simulink model "bille_synthese_RST"  (R2019a)
settings: Solver=VariableStepAuto  StartTime=0.0  StopTime=20  RelTol=1e-3
values from neighbouring files (symbols this model uses):
  f = 7E-5    (= 7e-05)    [BallOnBeam.m]
  J = 4.6E-5    (= 4.6e-05)    [BallOnBeam.m]
  k = 0.026    [BallOnBeam.m]
  k1 = 7    [BallOnBeam.m]
  k2 = 28.65    [BallOnBeam.m]
  k3 = 0.0159    [BallOnBeam.m]
  kb = 6.1    [BallOnBeam.m]
  ki = 1.6    [BallOnBeam.m]
  kp = nm*J*wndes^2/(k2*k*ki)    (= 27.0462934428)    [BallOnBeam.m]
  kpi = rm*tii*ki/taudesi    (= 1.6)    [BallOnBeam.m]
  kv = (2*xides*J*wndes - f)/(kp*ki*k*k3)    (= 0.093347474441)    [BallOnBeam.m]
  lm = 0.001    [BallOnBeam.m]
  nm = 960    [BallOnBeam.m]
  r0 = x(3)    [BallOnBeam.m]
  r1 = x(4)    [BallOnBeam.m]
  r2 = x(5)    [BallOnBeam.m]
  rm = 0.33    [BallOnBeam.m]
  s1 = x(2)    [BallOnBeam.m]
  T = r0 + r1 + r2    [BallOnBeam.m]
  Te = 0.2    [BallOnBeam.m]
  tii = 0.5*lm/rm    (= 0.00151515151515)    [BallOnBeam.m]
settings Model: Creator=DELL  LastModifiedBy=DELL

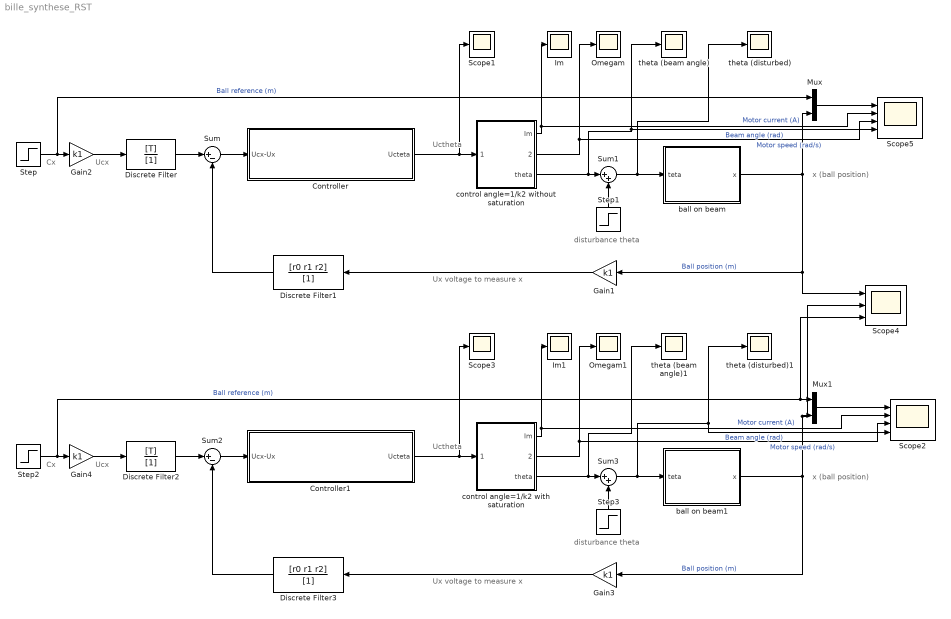
== system bille_synthese_RST ==
  note: disturbance theta
  note: Uctheta
  note: Ux voltage to measure x
  note: x (ball position)
  note: Cx
  note: Ucx
  note: Ux voltage to measure x
  note: Cx
  note: Uctheta
  note: Ucx
  note: disturbance theta
  note: x (ball position)
  Controller : Subsystem
  Controller1 : Subsystem
  Discrete Filter : DiscreteFilter  Numerator=[T]  Denominator=[1]
  Discrete Filter1 : DiscreteFilter  Numerator=[r0 r1 r2]  Denominator=[1]
  Discrete Filter2 : DiscreteFilter  Numerator=[T]  Denominator=[1]
  Discrete Filter3 : DiscreteFilter  Numerator=[r0 r1 r2]  Denominator=[1]
  Gain{1..4} (4 alike) : Gain  Gain=k1  SaturateOnIntegerOverflow=on  OutDataTypeStr=Inherit: Same as input  ParamDataTypeStr=Inherit: Same as input
  Im : Scope
  Im1 : Scope
  Mux : Mux  Inputs=2
  Mux1 : Mux  Inputs=2
  Omegam : Scope
  Omegam1 : Scope
  Scope1 : Scope
  Scope2 : Scope  NumInputPorts=4
  Scope3 : Scope
  Scope4 : Scope  NumInputPorts=3
  Scope5 : Scope  NumInputPorts=4
  Step : Step  After=0.1  SampleTime=0
  Step1 : Step  Time=10  After=1*pi/180  SampleTime=0
  Step2 : Step  After=0.1  SampleTime=0
  Step3 : Step  Time=10  After=1*pi/180  SampleTime=0
  Sum : Sum  Inputs=|+-  SaturateOnIntegerOverflow=on  InputSameDT=on  OutDataTypeStr=Inherit: Same as first input
  Sum1 : Sum  Inputs=|++  SaturateOnIntegerOverflow=on  InputSameDT=on  OutDataTypeStr=Inherit: Same as first input
  Sum2 : Sum  Inputs=|+-  SaturateOnIntegerOverflow=on  InputSameDT=on  OutDataTypeStr=Inherit: Same as first input
  Sum3 : Sum  Inputs=|++  SaturateOnIntegerOverflow=on  InputSameDT=on  OutDataTypeStr=Inherit: Same as first input
  ball on beam : Subsystem
  ball on beam1 : Subsystem
  control angle=1/k2 with saturation : Subsystem
  "control angle=1/k2 without saturation " : Subsystem
  theta (beam angle) : Scope
  theta (beam angle)1 : Scope
  theta (disturbed) : Scope
  theta (disturbed)1 : Scope
  wires:
  Sum1/1 -> theta (disturbed)/1, ball on beam/1(teta)
  "control angle=1/k2 without saturation "/2(omega) -> Omegam/1, Scope5/3  "Motor speed (rad/s)"
  Mux/1 -> Scope5/1
  "control angle=1/k2 without saturation "/3(theta) -> theta (beam angle)/1, Scope5/4, Sum1/1  "Beam angle (rad)"
  Step1/1 -> Sum1/2
  ball on beam/1(x) -> Scope4/1, Gain1/1, Mux/2  "Ball position (m)"
  Gain2/1 -> Discrete Filter/1
  Step/1 -> Mux/1, Gain2/1  "Ball reference (m)"
  Gain1/1 -> Discrete Filter1/1
  "control angle=1/k2 without saturation "/1(Im) -> Im/1, Scope5/2  "Motor current (A)"
  Discrete Filter/1 -> Sum/1
  Discrete Filter1/1 -> Sum/2
  Sum/1 -> Controller/1(Ucx-Ux)
  Controller/1(Ucteta) -> Scope1/1, "control angle=1/k2 without saturation "/1(Uctheta)
  control angle=1/k2 with saturation/3(theta) -> theta (beam angle)1/1, Sum3/1
  Sum2/1 -> Controller1/1(Ucx-Ux)
  Step3/1 -> Sum3/2
  Controller1/1(Ucteta) -> Scope3/1, control angle=1/k2 with saturation/1(Uctheta)
  Step2/1 -> Scope4/3, Mux1/1, Gain4/1  "Ball reference (m)"
  ball on beam1/1(x) -> Gain3/1, Scope4/2, Mux1/2  "Ball position (m)"
  Mux1/1 -> Scope2/1
  Sum3/1 -> theta (disturbed)1/1, Scope2/4, ball on beam1/1(teta)  "Beam angle (rad)"
  Discrete Filter3/1 -> Sum2/2
  Gain4/1 -> Discrete Filter2/1
  Gain3/1 -> Discrete Filter3/1
  control angle=1/k2 with saturation/2(omega) -> Omegam1/1, Scope2/3  "Motor speed (rad/s)"
  Discrete Filter2/1 -> Sum2/1
  control angle=1/k2 with saturation/1(Im) -> Im1/1, Scope2/2  "Motor current (A)"

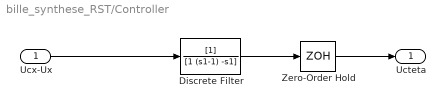
== system bille_synthese_RST/Controller ==
  Ucx-Ux : Inport
  Discrete Filter : DiscreteFilter  Denominator=[1 (s1-1) -s1]  SampleTime=Te
  Zero-Order Hold : ZeroOrderHold  SampleTime=-1
  Ucteta : Outport
  wires:
  Zero-Order Hold/1 -> Ucteta/1
  Discrete Filter/1 -> Zero-Order Hold/1
  Ucx-Ux/1 -> Discrete Filter/1

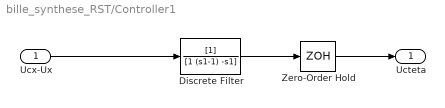
== system bille_synthese_RST/Controller1 ==
  Ucx-Ux : Inport
  Discrete Filter : DiscreteFilter  Denominator=[1 (s1-1) -s1]  SampleTime=Te
  Zero-Order Hold : ZeroOrderHold  SampleTime=-1
  Ucteta : Outport
  wires:
  Zero-Order Hold/1 -> Ucteta/1
  Discrete Filter/1 -> Zero-Order Hold/1
  Ucx-Ux/1 -> Discrete Filter/1

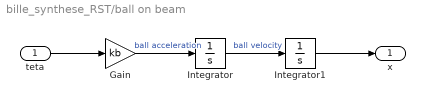
== system bille_synthese_RST/ball on beam ==
  teta : Inport
  Gain : Gain  Gain=kb
  Integrator : Integrator
  Integrator1 : Integrator
  x : Outport
  wires:
  Integrator/1 -> Integrator1/1  "ball velocity"
  Integrator1/1 -> x/1
  teta/1 -> Gain/1
  Gain/1 -> Integrator/1  "ball acceleration"

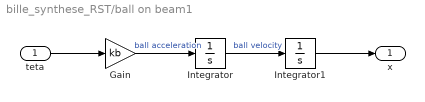
== system bille_synthese_RST/ball on beam1 ==
  teta : Inport
  Gain : Gain  Gain=kb
  Integrator : Integrator
  Integrator1 : Integrator
  x : Outport
  wires:
  Integrator/1 -> Integrator1/1  "ball velocity"
  Integrator1/1 -> x/1
  teta/1 -> Gain/1
  Gain/1 -> Integrator/1  "ball acceleration"

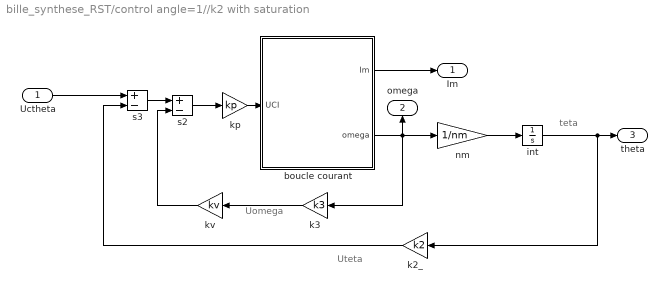
== system bille_synthese_RST/control angle=1//k2 with saturation ==
  note: Uomega
  note: teta
  note: Uteta
  Uctheta : Inport
  boucle courant : Subsystem
  int : Integrator
  k2_ : Gain  Gain=k2  SaturateOnIntegerOverflow=on  OutDataTypeStr=Inherit: Same as input  ParamDataTypeStr=Inherit: Same as input
  k3 : Gain  Gain=k3  SaturateOnIntegerOverflow=on  OutDataTypeStr=Inherit: Same as input  ParamDataTypeStr=Inherit: Same as input
  kp : Gain  Gain=kp  SaturateOnIntegerOverflow=on  OutDataTypeStr=Inherit: Same as input  ParamDataTypeStr=Inherit: Same as input
  kv : Gain  Gain=kv  SaturateOnIntegerOverflow=on  OutDataTypeStr=Inherit: Same as input  ParamDataTypeStr=Inherit: Same as input
  nm : Gain  Gain=1/nm  SaturateOnIntegerOverflow=on  OutDataTypeStr=Inherit: Same as input  ParamDataTypeStr=Inherit: Same as input
  s2 : Sum  Inputs=+-  SaturateOnIntegerOverflow=on  InputSameDT=on  OutDataTypeStr=Inherit: Same as first input
  s3 : Sum  Inputs=+-  SaturateOnIntegerOverflow=on  InputSameDT=on  OutDataTypeStr=Inherit: Same as first input
  Im : Outport
  omega : Outport  Port=2
  theta : Outport  Port=3
  wires:
  kp/1 -> boucle courant/1(UCI)
  s2/1 -> kp/1
  s3/1 -> s2/1
  nm/1 -> int/1
  boucle courant/2(omega) -> nm/1, k3/1, omega/1
  k3/1 -> kv/1
  kv/1 -> s2/2
  int/1 -> k2_/1, theta/1
  k2_/1 -> s3/2
  boucle courant/1(Im) -> Im/1
  Uctheta/1 -> s3/1

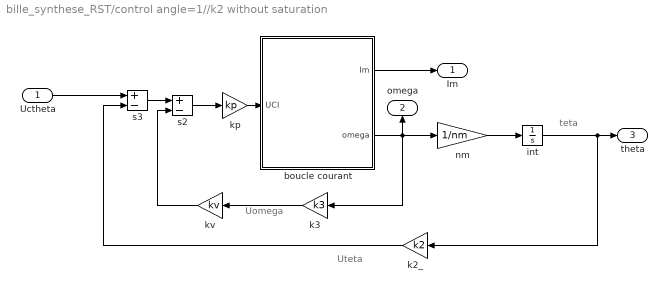
== system bille_synthese_RST/control angle=1//k2 without saturation  ==
  note: Uomega
  note: teta
  note: Uteta
  Uctheta : Inport
  boucle courant : Subsystem
  int : Integrator
  k2_ : Gain  Gain=k2  SaturateOnIntegerOverflow=on  OutDataTypeStr=Inherit: Same as input  ParamDataTypeStr=Inherit: Same as input
  k3 : Gain  Gain=k3  SaturateOnIntegerOverflow=on  OutDataTypeStr=Inherit: Same as input  ParamDataTypeStr=Inherit: Same as input
  kp : Gain  Gain=kp  SaturateOnIntegerOverflow=on  OutDataTypeStr=Inherit: Same as input  ParamDataTypeStr=Inherit: Same as input
  kv : Gain  Gain=kv  SaturateOnIntegerOverflow=on  OutDataTypeStr=Inherit: Same as input  ParamDataTypeStr=Inherit: Same as input
  nm : Gain  Gain=1/nm  SaturateOnIntegerOverflow=on  OutDataTypeStr=Inherit: Same as input  ParamDataTypeStr=Inherit: Same as input
  s2 : Sum  Inputs=+-  SaturateOnIntegerOverflow=on  InputSameDT=on  OutDataTypeStr=Inherit: Same as first input
  s3 : Sum  Inputs=+-  SaturateOnIntegerOverflow=on  InputSameDT=on  OutDataTypeStr=Inherit: Same as first input
  Im : Outport
  omega : Outport  Port=2
  theta : Outport  Port=3
  wires:
  kp/1 -> boucle courant/1(UCI)
  s2/1 -> kp/1
  s3/1 -> s2/1
  nm/1 -> int/1
  boucle courant/2(omega) -> nm/1, k3/1, omega/1
  k3/1 -> kv/1
  kv/1 -> s2/2
  int/1 -> k2_/1, theta/1
  k2_/1 -> s3/2
  boucle courant/1(Im) -> Im/1
  Uctheta/1 -> s3/1

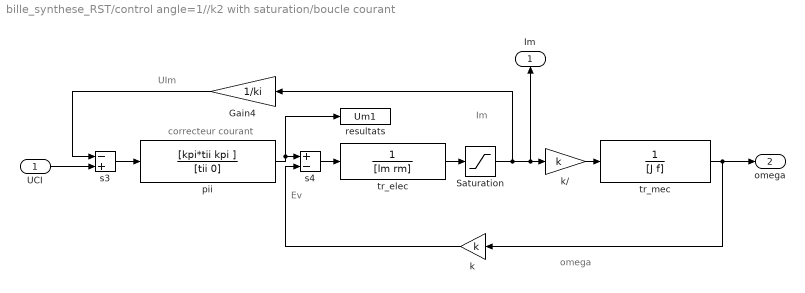
== system bille_synthese_RST/control angle=1//k2 with saturation/boucle courant ==
  note: correcteur courant
  note: Im
  note: Ev
  note: UIm
  note: omega
  UCI : Inport
  Gain4 : Gain  Gain=1/ki  SaturateOnIntegerOverflow=on  OutDataTypeStr=Inherit: Same as input  ParamDataTypeStr=Inherit: Same as input
  Saturation : Saturate  UpperLimit=16  LowerLimit=-16
  k : Gain  Gain=k  SaturateOnIntegerOverflow=on  OutDataTypeStr=Inherit: Same as input  ParamDataTypeStr=Inherit: Same as input
  "k/ " : Gain  Gain=k  SaturateOnIntegerOverflow=on  OutDataTypeStr=Inherit: Same as input  ParamDataTypeStr=Inherit: Same as input
  pii : TransferFcn  Numerator=[kpi*tii kpi ]  Denominator=[tii 0]
  resultats : ToWorkspace  VariableName=Um1
      settings: MaxDataPoints=20000
  s3 : Sum  Inputs=-+  SaturateOnIntegerOverflow=on  InputSameDT=on  OutDataTypeStr=Inherit: Same as first input
  s4 : Sum  Inputs=+-  SaturateOnIntegerOverflow=on  InputSameDT=on  OutDataTypeStr=Inherit: Same as first input
  tr_elec : TransferFcn  Denominator=[lm rm]
  tr_mec : TransferFcn  Denominator=[J f]
  Im : Outport
  omega : Outport  Port=2
  wires:
  s4/1 -> tr_elec/1
  Gain4/1 -> s3/1
  s3/1 -> pii/1
  k/1 -> s4/2
  "k/ "/1 -> tr_mec/1
  tr_mec/1 -> k/1, omega/1
  UCI/1 -> s3/2
  pii/1 -> s4/1, resultats/1
  tr_elec/1 -> Saturation/1
  Saturation/1 -> Gain4/1, Im/1, "k/ "/1

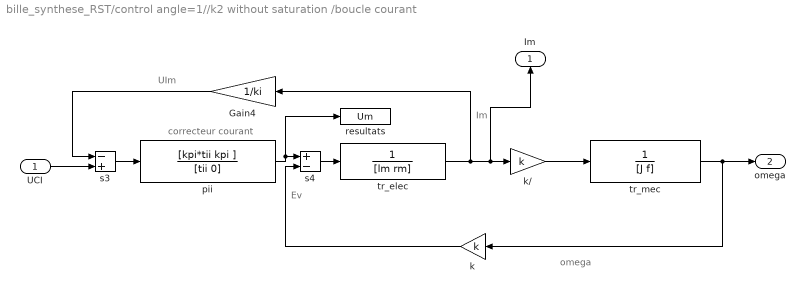
== system bille_synthese_RST/control angle=1//k2 without saturation /boucle courant ==
  note: correcteur courant
  note: Im
  note: Ev
  note: UIm
  note: omega
  UCI : Inport
  Gain4 : Gain  Gain=1/ki  SaturateOnIntegerOverflow=on  OutDataTypeStr=Inherit: Same as input  ParamDataTypeStr=Inherit: Same as input
  k : Gain  Gain=k  SaturateOnIntegerOverflow=on  OutDataTypeStr=Inherit: Same as input  ParamDataTypeStr=Inherit: Same as input
  "k/ " : Gain  Gain=k  SaturateOnIntegerOverflow=on  OutDataTypeStr=Inherit: Same as input  ParamDataTypeStr=Inherit: Same as input
  pii : TransferFcn  Numerator=[kpi*tii kpi ]  Denominator=[tii 0]
  resultats : ToWorkspace  VariableName=Um
      settings: MaxDataPoints=20000
  s3 : Sum  Inputs=-+  SaturateOnIntegerOverflow=on  InputSameDT=on  OutDataTypeStr=Inherit: Same as first input
  s4 : Sum  Inputs=+-  SaturateOnIntegerOverflow=on  InputSameDT=on  OutDataTypeStr=Inherit: Same as first input
  tr_elec : TransferFcn  Denominator=[lm rm]
  tr_mec : TransferFcn  Denominator=[J f]
  Im : Outport
  omega : Outport  Port=2
  wires:
  s4/1 -> tr_elec/1
  Gain4/1 -> s3/1
  s3/1 -> pii/1
  k/1 -> s4/2
  "k/ "/1 -> tr_mec/1
  tr_mec/1 -> k/1, omega/1
  UCI/1 -> s3/2
  pii/1 -> s4/1, resultats/1
  tr_elec/1 -> Gain4/1, "k/ "/1, Im/1
